simulink model "ArtUrban_energyCalc"  (R2021a)
settings: Solver=FixedStepAuto  StartTime=0.0  StopTime=1231  FixedStep=1  RelTol=1e-3
values from neighbouring files (symbols this model uses):
  A = 1.6    [vehParam.m]
  Cd = 0.6    [vehParam.m]
  f = 0.012    [vehParam.m]
  g = 9.8    [vehParam.m]
  mass = 650    [vehParam.m]
  rho = 1.2    [vehParam.m]
libraries: simulink x1
settings Model: Creator=asus  LastModifiedBy=asus

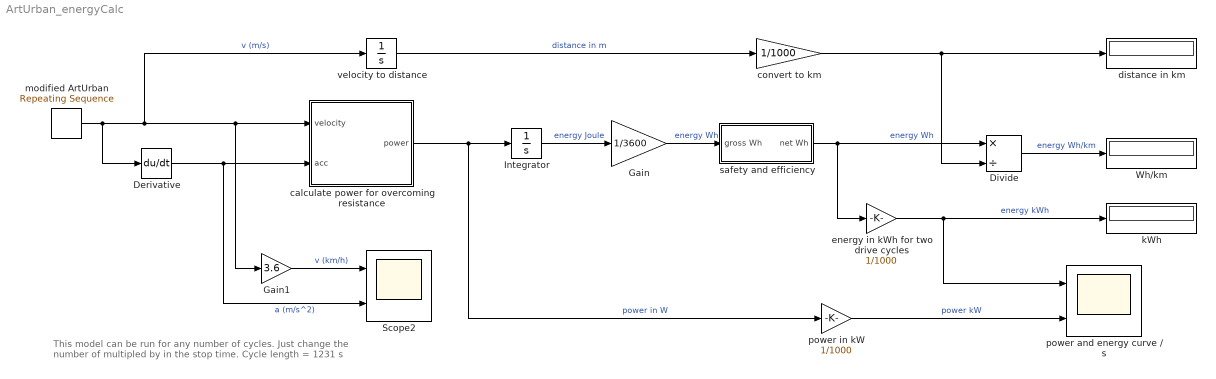
== system ArtUrban_energyCalc ==
  note: This model can be run for any number of cycles. Just change the number of multipled by in the stop time. Cycle length = 1231 s
  Derivative : Derivative
  Divide : Product  Inputs=*/
  Gain : Gain  Gain=1/3600
  Gain1 : Gain  Gain=3.6
  Integrator : Integrator
  Scope2 : Scope  NumInputPorts=2
  Wh/km : Display
  calculate power for overcoming resistance : Subsystem
  convert to km : Gain  Gain=1/1000
  distance in km : Display
  energy in kWh for two drive cycles : Gain  Gain=1/1000
  kWh : Display
  modified ArtUrban : simulink/Sources/Repeating Sequence  rep_seq_t=time_DriveCycle  rep_seq_y=vel_DriveCycle
  power and energy curve / s : Scope  NumInputPorts=2
  power in kW : Gain  Gain=1/1000
  safety and efficiency : Subsystem
  velocity to distance : Integrator
  wires:
  velocity to distance/1 -> convert to km/1  "distance in m"
  calculate power for overcoming resistance/1(power) -> power in kW/1, Integrator/1  "power in W"
  modified ArtUrban/1 -> velocity to distance/1, Gain1/1, calculate power for overcoming resistance/1(velocity), Derivative/1  "v (m/s)"
  energy in kWh for two drive cycles/1 -> power and energy curve / s/1, kWh/1  "energy kWh"
  Gain/1 -> safety and efficiency/1(gross Wh)  "energy Wh"
  Integrator/1 -> Gain/1  "energy Joule"
  power in kW/1 -> power and energy curve / s/2  "power kW"
  Gain1/1 -> Scope2/1  "v (km/h)"
  convert to km/1 -> Divide/2, distance in km/1
  safety and efficiency/1(net Wh) -> Divide/1, energy in kWh for two drive cycles/1  "energy Wh"
  Derivative/1 -> calculate power for overcoming resistance/2(acc), Scope2/2  "a (m/s^2)"
  Divide/1 -> Wh/km/1  "energy Wh/km"

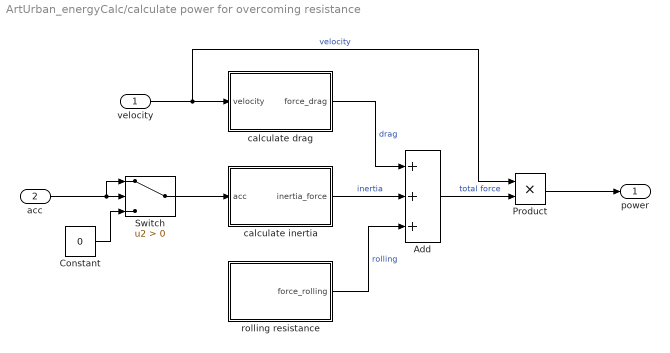
== system ArtUrban_energyCalc/calculate power for overcoming resistance ==
  velocity : Inport
  acc : Inport  Port=2
  Add : Sum  Inputs=+++
  Constant : Constant  Value=0
  Product : Product
  Switch : Switch  Criteria=u2 > Threshold
  calculate drag : Subsystem
  calculate inertia : Subsystem
  rolling resistance : Subsystem
  power : Outport
  wires:
  calculate drag/1(force_drag) -> Add/1  "drag"
  Add/1 -> Product/2  "total force"
  calculate inertia/1(inertia_force) -> Add/2  "inertia"
  rolling resistance/1(force_rolling) -> Add/3  "rolling"
  acc/1 -> Switch/1, Switch/2
  velocity/1 -> calculate drag/1(velocity), Product/1  "velocity"
  Product/1 -> power/1
  Constant/1 -> Switch/3
  Switch/1 -> calculate inertia/1(acc)

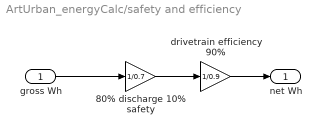
== system ArtUrban_energyCalc/safety and efficiency ==
  gross Wh : Inport
  80% discharge 10% safety : Gain  Gain=1/0.7
  drivetrain efficiency 90% : Gain  Gain=1/0.9
  net Wh : Outport
  wires:
  80% discharge 10% safety/1 -> drivetrain efficiency 90%/1
  drivetrain efficiency 90%/1 -> net Wh/1
  gross Wh/1 -> 80% discharge 10% safety/1

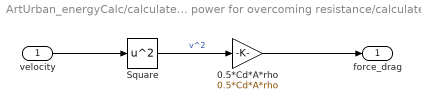
== system ArtUrban_energyCalc/calculate power for overcoming resistance/calculate drag ==
  velocity : Inport
  0.5*Cd*A*rho : Gain  Gain=0.5*Cd*A*rho
  Square : Math  Operator=square  SaturateOnIntegerOverflow=on
  force_drag : Outport
  wires:
  velocity/1 -> Square/1
  0.5*Cd*A*rho/1 -> force_drag/1
  Square/1 -> 0.5*Cd*A*rho/1  "v^2"

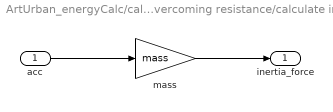
== system ArtUrban_energyCalc/calculate power for overcoming resistance/calculate inertia ==
  acc : Inport
  mass : Gain  Gain=mass
  inertia_force : Outport
  wires:
  mass/1 -> inertia_force/1
  acc/1 -> mass/1

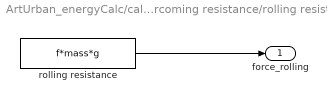
== system ArtUrban_energyCalc/calculate power for overcoming resistance/rolling resistance ==
  rolling resistance : Constant  Value=f*mass*g
  force_rolling : Outport
  wires:
  rolling resistance/1 -> force_rolling/1
